simulink model "Reactor_Gp2"  (Simulink 7.5)
settings: Solver=ode4  StartTime=0.0  StopTime=30.0  FixedStep=0.01  RelTol=1e-3
values from neighbouring files (symbols this model uses):
  K = 0.3199    [Ex14Gp1.m]    (also in Ex14Gp2.m)
  Kc = 1/K*(a1*(L/T)^b1+c1)    [Jrd3Deg_PID1tuning.m]    (also in Jrd3Degd_PID1tuning.m; MaxSenPID.m = pid(1))
  Ln = 0.5289    [Ex14Gp1.m]    (also in Ex14Gp2.m)
  T = 0.6238    [Ex14Gp1.m]    (also in Ex14Gp2.m)
  Td = T*(a3*(L/T)^b3+c3)    [Jrd3Deg_PID1tuning.m]    (also in Jrd3Degd_PID1tuning.m; MaxSenPID.m = pid(3))
  Ti = T*(a2*(L/T)^b2+c2)    [Jrd3Deg_PID1tuning.m]    (also in Jrd3Degd_PID1tuning.m; MaxSenPID.m = pid(2))
settings Model: Creator=Orlo  LastModifiedBy=oarrieta
settings OptimizationCC: InlineInvariantSignals=on  InitFltsAndDblsToZero=on
settings DebuggingCC: SaveWithParameterizedLinksMsg=none  SignalResolutionControl=TryResolveAllWithWarning  MultiTaskDSMMsg=warning  MultiTaskCondExecSysMsg=none  StrictBusMsg=None
settings RTWCC: IncludeERTFirstTime=on
settings GRTTargetCC: TargetFcnLib=ansi_tfl_tmw.mat

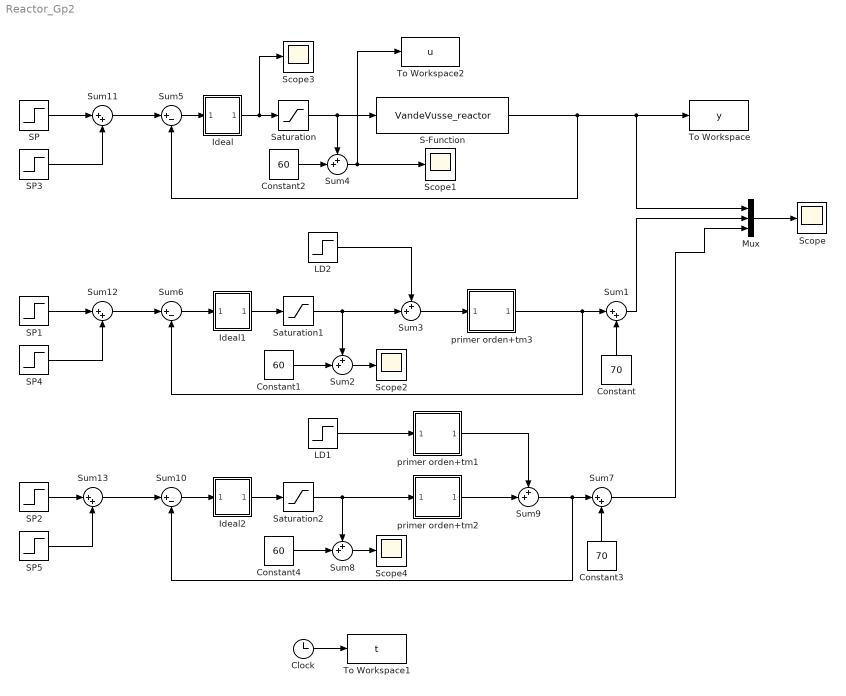
== system Reactor_Gp2 ==
  Clock : Clock
      settings: Decimation=10
  Constant : Constant  Value=70  OutDataType=sfix(16)  OutScaling=2^0
  Constant1 : Constant  Value=60  OutDataType=sfix(16)  OutScaling=2^0
  Constant2 : Constant  Value=60  OutDataType=sfix(16)  OutScaling=2^0
  Constant3 : Constant  Value=70  OutDataType=sfix(16)  OutScaling=2^0
  Constant4 : Constant  Value=60  OutDataType=sfix(16)  OutScaling=2^0
  Ideal : Subsystem  AncestorBlock=simulink_extras/Additional Linear/PID Controller  mask(Controlador PID Ideal){Kp=Kc, Ti=Ti, Td=Td, N=10}
      mask prompts: Kp "Ganancia Proporcional"; Ti "Tiempo Integral"; Td "Tiempo Derivativo"; N "Filtro"
      mask help:
      | Introduzca los valores para la Ganancia Proporcional Kp, el Tiempo Integral Ti y el Tiempo Derivativo Td
      | Kp[1+1/Tis+Tds/(1+Td/Ns)]
      mask Help: This block implements a PID controller where parameters are entered for the Proportional, Integral and Derivative terms. Unmask this block to see how it works. The derivative term is implemented using a true derivative block.
      mask Display: disp('PID')
  Ideal1 : Subsystem  AncestorBlock=simulink_extras/Additional Linear/PID Controller  mask(Controlador PID Ideal){Kp=Kc, Ti=Ti, Td=Td, N=10}
      mask prompts: Kp "Ganancia Proporcional"; Ti "Tiempo Integral"; Td "Tiempo Derivativo"; N "Filtro"
      mask help:
      | Introduzca los valores para la Ganancia Proporcional Kp, el Tiempo Integral Ti y el Tiempo Derivativo Td
      | Kp[1+1/Tis+Tds/(1+Td/Ns)]
      mask Help: This block implements a PID controller where parameters are entered for the Proportional, Integral and Derivative terms. Unmask this block to see how it works. The derivative term is implemented using a true derivative block.
      mask Display: disp('PID')
  Ideal2 : Subsystem  AncestorBlock=simulink_extras/Additional Linear/PID Controller  mask(Controlador PID Ideal){Kp=Kc, Ti=Ti, Td=Td, N=10}
      mask prompts: Kp "Ganancia Proporcional"; Ti "Tiempo Integral"; Td "Tiempo Derivativo"; N "Filtro"
      mask help:
      | Introduzca los valores para la Ganancia Proporcional Kp, el Tiempo Integral Ti y el Tiempo Derivativo Td
      | Kp[1+1/Tis+Tds/(1+Td/Ns)]
      mask Help: This block implements a PID controller where parameters are entered for the Proportional, Integral and Derivative terms. Unmask this block to see how it works. The derivative term is implemented using a true derivative block.
      mask Display: disp('PID')
  LD1 : Step  Time=10  SampleTime=0
  LD2 : Step  Time=10  SampleTime=0
  Mux : Mux  Inputs=3
  S-Function : S-Function  FunctionName=VandeVusse_reactor  Parameters=2.9175, 1.10  EnableBusSupport=off
  SP : Step  Before=70  After=60  SampleTime=0
  SP1 : Step  After=-10  SampleTime=0
  SP2 : Step  After=-10  SampleTime=0
  SP3 : Step  Time=20  After=5  SampleTime=0
  SP4 : Step  Time=20  After=5  SampleTime=0
  SP5 : Step  Time=20  After=5  SampleTime=0
  Saturation : Saturate  UpperLimit=40  LowerLimit=-60
  Saturation1 : Saturate  UpperLimit=40  LowerLimit=-60
  Saturation2 : Saturate  UpperLimit=40  LowerLimit=-60
  Scope{,1..4} (5 alike) : Scope
      Scope settings: YMin=54  YMax=74
      Scope1 settings: YMin=77  YMax=97
      Scope2 settings: YMin=65  YMax=90  SaveName=ScopeData2
      Scope3 settings: YMin=87.6517  YMax=87.6518  SaveName=ScopeData3
      Scope4 settings: YMin=65  YMax=90  SaveName=ScopeData4
  Sum{1,7,11..13} (5 alike) : Sum  Inputs=|++  OutDataType=sfix(16)  OutScaling=2^0  SaturateOnIntegerOverflow=on
  Sum10 : Sum  Inputs=|+-  OutDataType=sfix(16)  OutScaling=2^0  SaturateOnIntegerOverflow=on
  Sum{2..4,8..9} (5 alike) : Sum  Inputs=++|  OutDataType=sfix(16)  OutScaling=2^0  SaturateOnIntegerOverflow=on
  Sum5 : Sum  Inputs=|+-  OutDataType=sfix(16)  OutScaling=2^0  SaturateOnIntegerOverflow=on
  Sum6 : Sum  Inputs=|+-  OutDataType=sfix(16)  OutScaling=2^0  SaturateOnIntegerOverflow=on
  To Workspace : ToWorkspace  VariableName=y  SampleTime=-1  SaveFormat=Array
  To Workspace1 : ToWorkspace  VariableName=t  SampleTime=-1  SaveFormat=Array
  To Workspace2 : ToWorkspace  VariableName=u  SampleTime=-1  SaveFormat=Array
  primer orden+tm1 : Subsystem  mask(Modelo de primer orden mas tiempo muerto){K=5.4624, T=0.6829, L=0.2209}
      mask prompts: K "Ganancia"; T "Constante de tiempo"; L "Retardo"
      mask help:
      | Introduzca el valor para los parametros de la constante de tiempo y del retardo para el sistema de primer orden con retardo
      | Gm(s)=exp(-Ls)/(1+Ts)
      mask Display: disp('Modelo')
  primer orden+tm2 : Subsystem  mask(Modelo de primer orden mas tiempo muerto){K=K, T=T, L=Ln}
      mask prompts: K "Ganancia"; T "Constante de tiempo"; L "Retardo"
      mask help:
      | Introduzca el valor para los parametros de la constante de tiempo y del retardo para el sistema de primer orden con retardo
      | Gm(s)=exp(-Ls)/(1+Ts)
      mask Display: disp('Modelo')
  primer orden+tm3 : Subsystem  mask(Modelo de primer orden mas tiempo muerto){K=K, T=T, L=Ln}
      mask prompts: K "Ganancia"; T "Constante de tiempo"; L "Retardo"
      mask help:
      | Introduzca el valor para los parametros de la constante de tiempo y del retardo para el sistema de primer orden con retardo
      | Gm(s)=exp(-Ls)/(1+Ts)
      mask Display: disp('Modelo')
  wires:
  S-Function/1 -> Sum5/2, Mux/1, To Workspace/1
  Ideal/1(Out_1) -> Saturation/1, Scope3/1
  Saturation/1 -> S-Function/1, Sum4/1
  LD2/1 -> Sum3/1
  Saturation1/1 -> Sum2/1, Sum3/2
  Ideal1/1(Out_1) -> Saturation1/1
  Constant/1 -> Sum1/2
  Mux/1 -> Scope/1
  Sum1/1 -> Mux/2
  Sum2/1 -> Scope2/1
  Constant1/1 -> Sum2/2
  Sum4/1 -> Scope1/1, To Workspace2/1
  Constant2/1 -> Sum4/2
  Sum5/1 -> Ideal/1(In_1)
  Sum6/1 -> Ideal1/1(In_1)
  LD1/1 -> primer orden+tm1/1(In_1)
  primer orden+tm1/1(Out_1) -> Sum9/1
  primer orden+tm2/1(Out_1) -> Sum9/2
  Saturation2/1 -> Sum8/1, primer orden+tm2/1(In_1)
  Ideal2/1(Out_1) -> Saturation2/1
  Sum9/1 -> Sum7/1, Sum10/2
  Constant3/1 -> Sum7/2
  Sum8/1 -> Scope4/1
  Constant4/1 -> Sum8/2
  Sum10/1 -> Ideal2/1(In_1)
  Sum7/1 -> Mux/3
  Clock/1 -> To Workspace1/1
  SP/1 -> Sum11/1
  SP3/1 -> Sum11/2
  Sum11/1 -> Sum5/1
  SP1/1 -> Sum12/1
  Sum12/1 -> Sum6/1
  SP4/1 -> Sum12/2
  SP2/1 -> Sum13/1
  Sum13/1 -> Sum10/1
  SP5/1 -> Sum13/2
  primer orden+tm3/1(Out_1) -> Sum1/1, Sum6/2
  Sum3/1 -> primer orden+tm3/1(In_1)

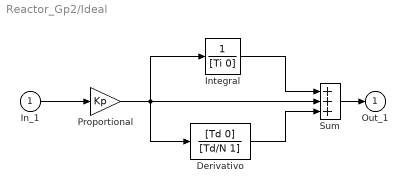
== system Reactor_Gp2/Ideal ==
  In_1 : Inport  OutDataType=sfix(16)  OutScaling=2^0
  Derivativo : TransferFcn  Numerator=[Td 0]  Denominator=[Td/N 1]
  Integral : TransferFcn  Denominator=[Ti 0]
  Proportional : Gain  Gain=Kp  ParameterDataType=sfix(16)  ParameterScaling=2^0  OutDataType=sfix(16)  OutScaling=2^0  SaturateOnIntegerOverflow=on  OutDataTypeStr=Inherit: Same as input  ParamDataTypeStr=Inherit: Same as input
  Sum : Sum  Inputs=+++  OutDataType=sfix(16)  OutScaling=2^0  SaturateOnIntegerOverflow=on  InputSameDT=on  OutDataTypeStr=Inherit: Same as first input
  Out_1 : Outport  OutDataType=sfix(16)  OutScaling=2^0  InitialOutput=0
  wires:
  Sum/1 -> Out_1/1
  In_1/1 -> Proportional/1
  Proportional/1 -> Sum/2, Integral/1, Derivativo/1
  Derivativo/1 -> Sum/3
  Integral/1 -> Sum/1

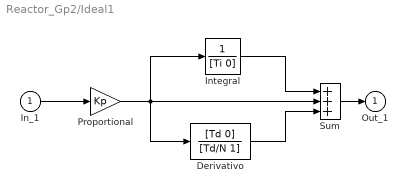
== system Reactor_Gp2/Ideal1 ==
  In_1 : Inport  OutDataType=sfix(16)  OutScaling=2^0
  Derivativo : TransferFcn  Numerator=[Td 0]  Denominator=[Td/N 1]
  Integral : TransferFcn  Denominator=[Ti 0]
  Proportional : Gain  Gain=Kp  ParameterDataType=sfix(16)  ParameterScaling=2^0  OutDataType=sfix(16)  OutScaling=2^0  SaturateOnIntegerOverflow=on  OutDataTypeStr=Inherit: Same as input  ParamDataTypeStr=Inherit: Same as input
  Sum : Sum  Inputs=+++  OutDataType=sfix(16)  OutScaling=2^0  SaturateOnIntegerOverflow=on  InputSameDT=on  OutDataTypeStr=Inherit: Same as first input
  Out_1 : Outport  OutDataType=sfix(16)  OutScaling=2^0  InitialOutput=0
  wires:
  Sum/1 -> Out_1/1
  In_1/1 -> Proportional/1
  Proportional/1 -> Sum/2, Integral/1, Derivativo/1
  Derivativo/1 -> Sum/3
  Integral/1 -> Sum/1

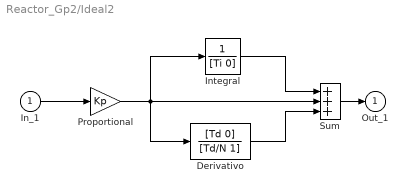
== system Reactor_Gp2/Ideal2 ==
  In_1 : Inport  OutDataType=sfix(16)  OutScaling=2^0
  Derivativo : TransferFcn  Numerator=[Td 0]  Denominator=[Td/N 1]
  Integral : TransferFcn  Denominator=[Ti 0]
  Proportional : Gain  Gain=Kp  ParameterDataType=sfix(16)  ParameterScaling=2^0  OutDataType=sfix(16)  OutScaling=2^0  SaturateOnIntegerOverflow=on  OutDataTypeStr=Inherit: Same as input  ParamDataTypeStr=Inherit: Same as input
  Sum : Sum  Inputs=+++  OutDataType=sfix(16)  OutScaling=2^0  SaturateOnIntegerOverflow=on  InputSameDT=on  OutDataTypeStr=Inherit: Same as first input
  Out_1 : Outport  OutDataType=sfix(16)  OutScaling=2^0  InitialOutput=0
  wires:
  Sum/1 -> Out_1/1
  In_1/1 -> Proportional/1
  Proportional/1 -> Sum/2, Integral/1, Derivativo/1
  Derivativo/1 -> Sum/3
  Integral/1 -> Sum/1

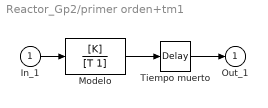
== system Reactor_Gp2/primer orden+tm1 ==
  In_1 : Inport  OutDataType=sfix(16)  OutScaling=2^0
  Modelo : TransferFcn  Numerator=[K]  Denominator=[T 1]
  Tiempo muerto : TransportDelay  DelayTime=L
  Out_1 : Outport  OutDataType=sfix(16)  OutScaling=2^0  InitialOutput=0
  wires:
  Modelo/1 -> Tiempo muerto/1
  In_1/1 -> Modelo/1
  Tiempo muerto/1 -> Out_1/1

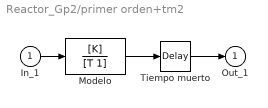
== system Reactor_Gp2/primer orden+tm2 ==
  In_1 : Inport  OutDataType=sfix(16)  OutScaling=2^0
  Modelo : TransferFcn  Numerator=[K]  Denominator=[T 1]
  Tiempo muerto : TransportDelay  DelayTime=L
  Out_1 : Outport  OutDataType=sfix(16)  OutScaling=2^0  InitialOutput=0
  wires:
  Modelo/1 -> Tiempo muerto/1
  In_1/1 -> Modelo/1
  Tiempo muerto/1 -> Out_1/1

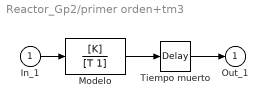
== system Reactor_Gp2/primer orden+tm3 ==
  In_1 : Inport  OutDataType=sfix(16)  OutScaling=2^0
  Modelo : TransferFcn  Numerator=[K]  Denominator=[T 1]
  Tiempo muerto : TransportDelay  DelayTime=L
  Out_1 : Outport  OutDataType=sfix(16)  OutScaling=2^0  InitialOutput=0
  wires:
  Modelo/1 -> Tiempo muerto/1
  In_1/1 -> Modelo/1
  Tiempo muerto/1 -> Out_1/1
